simulink model "ModeloTotal"  (R2023b)
settings: Solver=VariableStepAuto  StartTime=0.0  StopTime=10.0  RelTol=1e-3
settings Model: Creator=USUARIO  LastModifiedBy=USUARIO
settings DebuggingCC: ParameterOverflowMsg=none

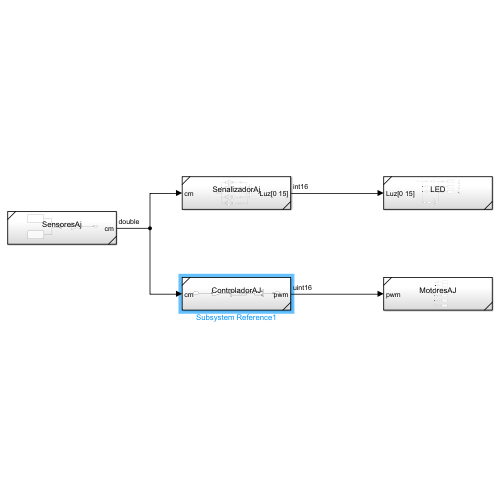
[thumbnail: Simulink's stored preview of the top-level diagram]
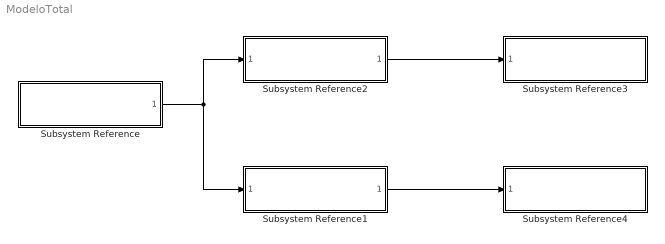
== system ModeloTotal ==
  Subsystem Reference : Subsystem  ReferencedSubsystem=SensoresAj
  Subsystem Reference1 : Subsystem  ReferencedSubsystem=ControladorAJ
  Subsystem Reference2 : Subsystem  ReferencedSubsystem=SenalizadorAj
  Subsystem Reference3 : Subsystem  ReferencedSubsystem=LED
  Subsystem Reference4 : Subsystem  ReferencedSubsystem=MotoresAJ
  wires:
  Subsystem Reference/1 -> Subsystem Reference1/1, Subsystem Reference2/1
  Subsystem Reference1/1 -> Subsystem Reference4/1
  Subsystem Reference2/1 -> Subsystem Reference3/1
